simulink model "ex3_sim1m"  (R2022b)
settings: Solver=ode45  StartTime=0.0  StopTime=2  MaxStep=0.0001  RelTol=1e-3
undefined symbols (not defined in the file): bit, d, denCd, denPc, denQd, denQdPd, numCd, numPc, numQd, numQdPd, r, Ts, umax
settings Model: Creator=loren  LastModifiedBy=loren
settings DataIOCC: ReturnWorkspaceOutputs=off

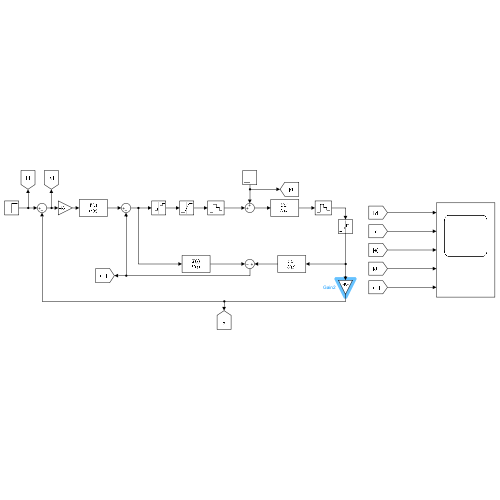
[thumbnail: Simulink's stored preview of the top-level diagram]
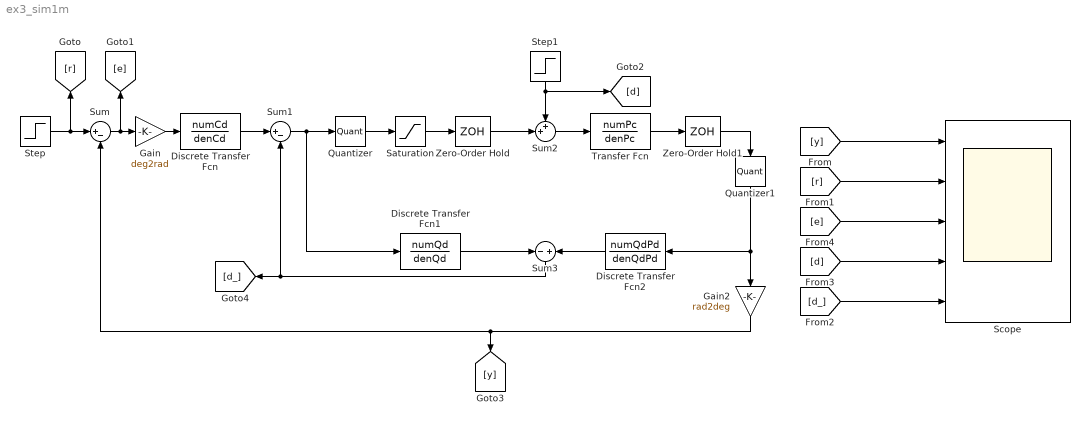
== system ex3_sim1m ==
  Discrete Transfer Fcn : DiscreteTransferFcn  Numerator=numCd  Denominator=denCd
  Discrete Transfer Fcn1 : DiscreteTransferFcn  Numerator=numQd  Denominator=denQd
  Discrete Transfer Fcn2 : DiscreteTransferFcn  Numerator=numQdPd  Denominator=denQdPd
  Gain : Gain  Gain=deg2rad
  Gain2 : Gain  Gain=rad2deg
  Quantizer : Quantizer  QuantizationInterval=2 * umax / 2^bit
  Quantizer1 : Quantizer  QuantizationInterval=pulse2rad
  Saturation : Saturate  UpperLimit=umax  LowerLimit=-umax
  Scope : Scope  NumInputPorts=5
  Step : Step  Time=r.t  After=r.A  SampleTime=0
  Step1 : Step  Time=d.t  After=d.A  SampleTime=0
  Sum : Sum  Inputs=|+-
  Sum1 : Sum  Inputs=|+-
  Sum2 : Sum  Inputs=++|
  Sum3 : Sum  Inputs=-|+
  Transfer Fcn : TransferFcn  Numerator=numPc  Denominator=denPc
  Zero-Order Hold : ZeroOrderHold  SampleTime=Ts
  Zero-Order Hold1 : ZeroOrderHold  SampleTime=Ts
  wires:
  Step/1 -> [r], Sum/1
  Discrete Transfer Fcn/1 -> Sum1/1
  Sum1/1 -> Discrete Transfer Fcn1/1, Quantizer/1
  Quantizer/1 -> Saturation/1
  Saturation/1 -> Zero-Order Hold/1
  Gain/1 -> Discrete Transfer Fcn/1
  Sum/1 -> [e], Gain/1
  Zero-Order Hold/1 -> Sum2/2
  Sum2/1 -> Transfer Fcn/1
  Zero-Order Hold1/1 -> Quantizer1/1
  Discrete Transfer Fcn1/1 -> Sum3/1
  Discrete Transfer Fcn2/1 -> Sum3/2
  Sum3/1 -> [d_], Sum1/2
  Transfer Fcn/1 -> Zero-Order Hold1/1
  Step1/1 -> Sum2/1, [d]
  [y] -> Scope/1
  [r] -> Scope/2
  [e] -> Scope/3
  [d] -> Scope/4
  [d_] -> Scope/5
  Quantizer1/1 -> Gain2/1, Discrete Transfer Fcn2/1
  Gain2/1 -> [y], Sum/2
